simulink model "levitatore_function"  (R2017a)
settings: Solver=VariableStepAuto  StartTime=0.0  StopTime=inf  RelTol=1e-3
values from neighbouring files (symbols this model uses):
  par = [m,km,R,L0,b,g]    [levitatoreMagnetico.m]    (also in temp1.mat = [0.2 19.62 50 0.5 0.1 9.81])
settings Model: Creator=Enrico Donato  LastModifiedBy=Enrico Donato

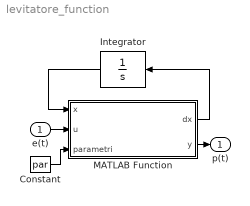
== system levitatore_function ==
  e(t) : Inport
  Constant : Constant  Value=par
  Integrator : Integrator  InitialCondition=zeros(3,1)
  MATLAB Function : MATLAB Function  TreatAsAtomicUnit=on
  p(t) : Outport
  wires:
  Constant/1 -> MATLAB Function/3(parametri)
  MATLAB Function/1(dx) -> Integrator/1
  Integrator/1 -> MATLAB Function/1(x)
  e(t)/1 -> MATLAB Function/2(u)
  MATLAB Function/2(y) -> p(t)/1

== matlab function levitatore_function/MATLAB Function ==
  data: x input; dx output; u input; y output; parametri input
function [dx,y] = fcn(x,u,parametri)
% Estrai i parametri dal terzo argomento della funzione.
m = parametri(1);
km = parametri(2);
R = parametri(3);
L = parametri(4);
b = parametri(5);
g = parametri(6);

% Definisci gli stati del modello (p,v,i).
p = x(1); v = x(2); i = x(3);

% Implementa la funzione generatrice f(x,u).
dp = v;
dv = g - (km/m)*(i/p)^2 - (b/m)*v^2;
di = (1/(L+(km/p)))*(-R*i + km*v*i/p^2 + u);

% Associa i valori alle uscite.
dx = [dp; dv; di];
y = p;
end
